simulink model "TireSimple"  (R2026b)
settings: Solver=ode45  StopTime=1
undefined symbols (not defined in the file): Tire
settings Model: DataDictionary=VehicleData.sldd  Creator=Xu Dingyi  LastModifiedBy=29358

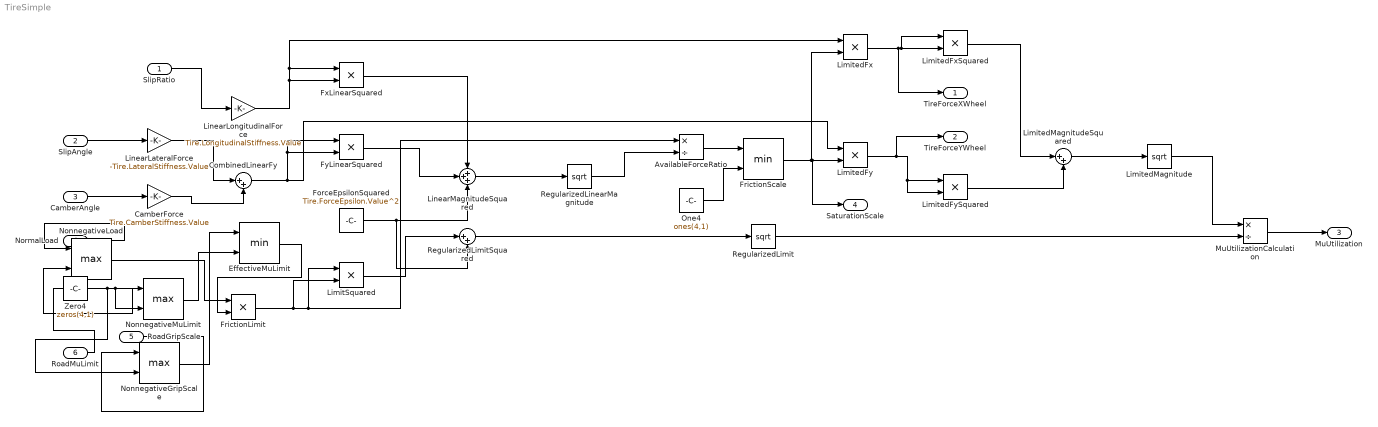
== system TireSimple ==
  SlipRatio : Inport  OutDataTypeStr=double  PortDimensions=[4 1]
  SlipAngle : Inport  Port=2  OutDataTypeStr=double  PortDimensions=[4 1]
  CamberAngle : Inport  Port=3  OutDataTypeStr=double  PortDimensions=[4 1]
  NormalLoad : Inport  Port=4  OutDataTypeStr=double  PortDimensions=[4 1]
  RoadGripScale : Inport  Port=5  OutDataTypeStr=double  PortDimensions=[4 1]
  RoadMuLimit : Inport  Port=6  PortDimensions=4
  AvailableForceRatio : Product  Inputs=*/
  CamberForce : Gain  Gain=Tire.CamberStiffness.Value
  CombinedLinearFy : Sum  Inputs=|++
  EffectiveMuLimit : MinMax  Inputs=2
  ForceEpsilonSquared : Constant  Value=Tire.ForceEpsilon.Value^2  OutDataTypeStr=double
  FrictionLimit : Product  Inputs=**
  FrictionScale : MinMax  Inputs=2
  FxLinearSquared : Product  Inputs=**
  FyLinearSquared : Product  Inputs=**
  LimitSquared : Product  Inputs=**
  LimitedFx : Product  Inputs=**
  LimitedFxSquared : Product  Inputs=**
  LimitedFy : Product  Inputs=**
  LimitedFySquared : Product  Inputs=**
  LimitedMagnitude : Sqrt
  LimitedMagnitudeSquared : Sum  Inputs=|++
  LinearLateralForce : Gain  Gain=-Tire.LateralStiffness.Value
  LinearLongitudinalForce : Gain  Gain=Tire.LongitudinalStiffness.Value
  LinearMagnitudeSquared : Sum  Inputs=+++
  MuUtilizationCalculation : Product  Inputs=*/
  NonnegativeGripScale : MinMax  Function=max  Inputs=2
  NonnegativeLoad : MinMax  Function=max  Inputs=2
  NonnegativeMuLimit : MinMax  Function=max  Inputs=2
  One4 : Constant  Value=ones(4,1)  OutDataTypeStr=double
  RegularizedLimit : Sqrt
  RegularizedLimitSquared : Sum  Inputs=|++
  RegularizedLinearMagnitude : Sqrt
  Zero4 : Constant  Value=zeros(4,1)  OutDataTypeStr=double
  TireForceXWheel : Outport
  TireForceYWheel : Outport  Port=2
  MuUtilization : Outport  Port=3
  SaturationScale : Outport  Port=4
  wires:
  MuUtilizationCalculation/1 -> MuUtilization/1
  RegularizedLimit/1 -> MuUtilizationCalculation/2
  LimitedMagnitude/1 -> MuUtilizationCalculation/1
  RegularizedLimitSquared/1 -> RegularizedLimit/1
  LimitSquared/1 -> RegularizedLimitSquared/1
  LimitedMagnitudeSquared/1 -> LimitedMagnitude/1
  LimitedFySquared/1 -> LimitedMagnitudeSquared/2
  LimitedFxSquared/1 -> LimitedMagnitudeSquared/1
  LimitedFy/1 -> LimitedFySquared/1, LimitedFySquared/2, TireForceYWheel/1
  LimitedFx/1 -> LimitedFxSquared/1, LimitedFxSquared/2, TireForceXWheel/1
  FrictionScale/1 -> LimitedFy/2, SaturationScale/1, LimitedFx/2
  One4/1 -> FrictionScale/2
  AvailableForceRatio/1 -> FrictionScale/1
  RegularizedLinearMagnitude/1 -> AvailableForceRatio/2
  LinearMagnitudeSquared/1 -> RegularizedLinearMagnitude/1
  ForceEpsilonSquared/1 -> LinearMagnitudeSquared/3, RegularizedLimitSquared/2
  FyLinearSquared/1 -> LinearMagnitudeSquared/2
  FxLinearSquared/1 -> LinearMagnitudeSquared/1
  CamberAngle/1 -> CamberForce/1
  SlipAngle/1 -> LinearLateralForce/1
  RoadGripScale/1 -> NonnegativeGripScale/1
  LinearLateralForce/1 -> CombinedLinearFy/1
  CamberForce/1 -> CombinedLinearFy/2
  CombinedLinearFy/1 -> FyLinearSquared/1, FyLinearSquared/2, LimitedFy/1
  NonnegativeLoad/1 -> FrictionLimit/1
  EffectiveMuLimit/1 -> FrictionLimit/2
  FrictionLimit/1 -> LimitSquared/1, AvailableForceRatio/1, LimitSquared/2
  SlipRatio/1 -> LinearLongitudinalForce/1
  LinearLongitudinalForce/1 -> FxLinearSquared/1, LimitedFx/1, FxLinearSquared/2
  NormalLoad/1 -> NonnegativeLoad/1
  Zero4/1 -> NonnegativeMuLimit/2, NonnegativeLoad/2, NonnegativeGripScale/2
  NonnegativeGripScale/1 -> EffectiveMuLimit/1
  RoadMuLimit/1 -> NonnegativeMuLimit/1
  NonnegativeMuLimit/1 -> EffectiveMuLimit/2
